simulink library "Scene_Systems"  (R2025b)
settings: Solver=VariableStepAuto  StartTime=0.0  StopTime=10.0  RelTol=1e-3
libraries: sm_car_scene_crg_custom x1, sm_car_scene_crg_custom_f x1, sm_car_scene_crg_hockenheim x1, sm_car_scene_crg_hockenheim_f x1, sm_car_scene_crg_kyalami x1, sm_car_scene_crg_kyalami_f x1, sm_car_scene_crg_mallory_park x1, sm_car_scene_crg_mallory_park_f x1, sm_car_scene_crg_nurburgring_n x1, sm_car_scene_crg_nurburgring_n_f x1, sm_car_scene_crg_pikes_peak x1, sm_car_scene_crg_plateau x1
Description:
  | Simscape Vehicle Templates Library
  | 
  | Copyright 2018-2024 The MathWorks, Inc.
settings Model: Creator=smiller  LastModifiedBy=smiller
settings ModelReferenceCC: EnableRefExpFcnMdlSchedulingChecks=on
settings RTWCC: GPUComputeCapability=3.5

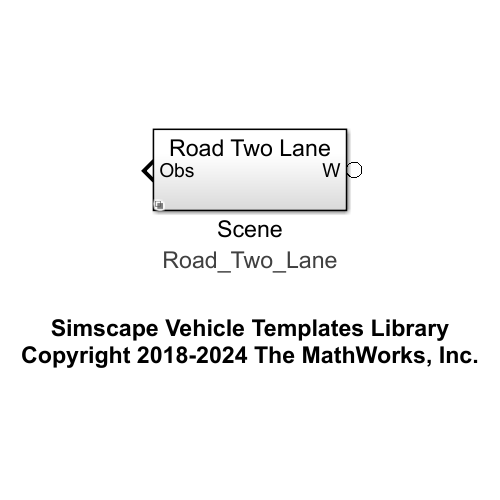
[thumbnail: Simulink's stored preview of the top-level diagram]
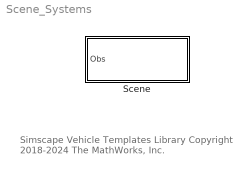
== system Scene_Systems ==
  note: Simscape Vehicle Templates Library
      | Copyright 2018-2024 The MathWorks, Inc.
  Scene : Subsystem  Variant=on  VariantControlMode=label  LabelModeActiveChoice=Road_Two_Lane
      settings: AttributesFormatString=%<LabelModeActiveChoice>

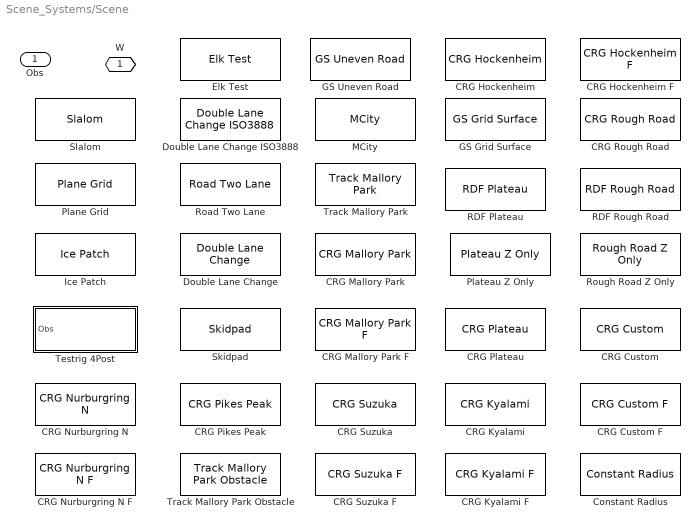
== system Scene_Systems/Scene ==
  CRG Custom : sm_car_scene_crg_custom/CRG Custom  VariantControl=CRG_Custom  geometry=Scene.CRG_Custom.Geometry
  CRG Custom F : sm_car_scene_crg_custom_f/CRG Custom F  VariantControl=CRG_Custom_F  geometry=Scene.CRG_Custom_F.Geometry
  CRG Hockenheim : sm_car_scene_crg_hockenheim/CRG Hockenheim  VariantControl=CRG_Hockenheim  geometry=Scene.CRG_Hockenheim.Geometry
  CRG Hockenheim F : sm_car_scene_crg_hockenheim_f/CRG Hockenheim F  VariantControl=CRG_Hockenheim_F  geometry=Scene.CRG_Hockenheim_F.Geometry
  CRG Kyalami : sm_car_scene_crg_kyalami/CRG Kyalami  VariantControl=CRG_Kyalami  geometry=Scene.CRG_Kyalami.Geometry
  CRG Kyalami F : sm_car_scene_crg_kyalami_f/CRG Kyalami F  VariantControl=CRG_Kyalami_F  geometry=Scene.CRG_Kyalami_F.Geometry
  CRG Mallory Park : sm_car_scene_crg_mallory_park/CRG Mallory Park  VariantControl=CRG_Mallory_Park  geometry=Scene.CRG_Mallory_Park.Geometry
  CRG Mallory Park F : sm_car_scene_crg_mallory_park_f/CRG Mallory Park F  VariantControl=CRG_Mallory_Park_F  geometry=Scene.CRG_Mallory_Park_F.Geometry
  CRG Nurburgring N : sm_car_scene_crg_nurburgring_n/CRG Nurburgring N  VariantControl=CRG_Nurburgring_N  geometry=Scene.CRG_Nurburgring_N.Geometry
  CRG Nurburgring N F : sm_car_scene_crg_nurburgring_n_f/CRG Nurburgring N F  VariantControl=CRG_Nurburgring_N_F  geometry=Scene.CRG_Nurburgring_N_F.Geometry
  CRG Pikes Peak : sm_car_scene_crg_pikes_peak/CRG Pikes Peak  VariantControl=CRG_Pikes_Peak  geometry=Scene.CRG_Pikes_Peak.Geometry
  CRG Plateau : sm_car_scene_crg_plateau/CRG Plateau  VariantControl=CRG_Plateau  geometry=Scene.CRG_Plateau.Geometry
  CRG Rough Road : sm_car_scene_crg_rough_road/CRG Rough Road  VariantControl=CRG_Rough_Road  geometry=Scene.CRG_Rough_Road.Geometry
  CRG Suzuka : sm_car_scene_crg_suzuka/CRG Suzuka  VariantControl=CRG_Suzuka  geometry=Scene.CRG_Suzuka.Geometry
  CRG Suzuka F : sm_car_scene_crg_suzuka_f/CRG Suzuka F  VariantControl=CRG_Suzuka_F  geometry=Scene.CRG_Suzuka_F.Geometry
  Constant Radius : sm_car_scene_constant_radius_cl/Constant Radius  VariantControl=Constant_Radius  circ_in=Scene.Constant_Radius_CL.Circle_Inner  circ_out=Scene.Constant_Radius_CL.Circle_Outer  plane=Scene.Constant_Radius_CL.Plane
  Double Lane Change : sm_car_scene_double_lane_change/Double Lane Change  VariantControl=Double_Lane_Change  road=Scene.Double_Lane_Change.Road  dashes=Scene.Double_Lane_Change.Dashes  cones=Scene.Double_Lane_Change.Cones
  Double Lane Change ISO3888 : sm_car_scene_double_lane_change_iso3888/Double Lane Change ISO3888  VariantControl=Double_Lane_Change_ISO3888  road=Scene.Double_Lane_Change_ISO3888.Road  dashes=Scene.Double_Lane_Change_ISO3888.Dashes  cones=Scene.Double_Lane_Change_ISO3888.Cones
  Elk Test : sm_car_scene_elk_test/Elk Test  VariantControl=Elk_Test  road=Scene.Elk_Test.Road  dashes=Scene.Elk_Test.Dashes  ice_patch=Scene.Elk_Test.Ice
  GS Grid Surface : sm_car_scene_gs_grid_surface/GS Grid Surface  VariantControl=GS_Grid_Surface  grid_surface=Scene.GS_Grid_Surface
  GS Uneven Road : sm_car_scene_gs_uneven_road/GS Uneven Road  VariantControl=GS_Uneven_Road  geometry=Scene.GS_Uneven_Road.Geometry
  Ice Patch : sm_car_scene_ice_patch/Ice Patch  VariantControl=Ice_Patch  plane=Scene.Ice_Patch.Plane  grid=Scene.Ice_Patch.Grid  ice=Scene.Ice_Patch.Ice
  MCity : sm_car_scene_mcity/MCity  VariantControl=MCity  geometry=Scene.MCity.Geometry
  Plane Grid : sm_car_scene_plane_grid/Plane Grid  VariantControl=Plane_Grid  plane=Scene.Plane_Grid.Plane  grid=Scene.Plane_Grid.Grid
  Plateau Z Only : Plateau_Z_Only/Plateau Z Only  VariantControl=Plateau_Z_Only  RDF_Polyline=Scene.RDF_Plateau
  RDF Plateau : sm_car_scene_rdf_plateau/RDF Plateau  VariantControl=RDF_Plateau  RDF_Polyline=Scene.RDF_Plateau
  RDF Rough Road : sm_car_scene_rdf_rough_road/RDF Rough Road  VariantControl=RDF_Rough_Road  RDF_Polyline=Scene.RDF_Rough_Road
  Road Two Lane : sm_car_scene_road_two_lane/Road Two Lane  VariantControl=Road_Two_Lane  road=Scene.Road_Two_Lane.Road  dashes=Scene.Road_Two_Lane.Dashes
  Rough Road Z Only : Rough_Road_Z_Only/Rough Road Z Only  VariantControl=Rough_Road_Z_Only  RDF_Polyline=Scene.RDF_Rough_Road
  Skidpad : sm_car_scene_skidpad/Skidpad  VariantControl=Skidpad  circ_in=Scene.Skidpad.Circle_Inner  circ_out=Scene.Skidpad.Circle_Outer  plane=Scene.Skidpad.Plane
  Slalom : sm_car_scene_slalom/Slalom  VariantControl=Slalom  road=Scene.Slalom.Road  dashes=Scene.Slalom.Dashes  cones=Scene.Slalom.Cones  vehTraj=Maneuver.Trajectory
  Testrig 4Post : Subsystem  VariantControl=Testrig_4_Post
  Track Mallory Park : sm_car_scene_track_mallory_park/Track Mallory Park  VariantControl=Track_Mallory_Park  track=Scene.Mallory_Park.Track
  Track Mallory Park Obstacle : sm_car_scene_track_mallory_park_obstacle/Track Mallory Park Obstacle  VariantControl=Track_Mallory_Park_Obstacle  scene_data=Scene.Mallory_Park_Obstacle
  W : PMIOPort  Side=Left
  Obs : Outport  VectorParamsAs1DForOutWhenUnconnected=off

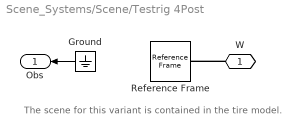
== system Scene_Systems/Scene/Testrig 4Post ==
  note: The scene for this variant is contained in the tire model.
  Ground : Ground
  Reference Frame : sm_lib/Frames and Transforms/Reference Frame
  W : PMIOPort  Side=Left
  Obs : Outport  VectorParamsAs1DForOutWhenUnconnected=off
  wires:
  Ground/1 -> Obs/1
  connections:
  W/RConn1 -- Reference Frame/RConn1
